simulink model "comparing_modell_MSfartoy"  (R2017b)
settings: Solver=ode45  StartTime=tstart  StopTime=tstop  RelTol=1e-3  EnableMultiTasking=on
values from neighbouring files (symbols this model uses):
  c = 0    [analyse_dynamics_v3.m]    (also in run_task_1_8.m = 1; system_identification.m = pid_matrix(i,:))
  den = data_matrix(i,2)    [system_identification.m]
  e_u_limit = 0.7    [parameters_speed_controller.m]    (also in run_task_1_8.m; system_identification.m = 100000)
  Ki_u = 0.08    [parameters_speed_controller.m]    (also in run_task_1_8.m; system_identification.m = c(4)*Ki_u_gain_list(i))
  Ki_u_est = c(4)*0.7    [system_identification.m]
  Kp_u = 80    [parameters_speed_controller.m]    (also in run_task_1_8.m; system_identification.m)
  Kp_u_est = c(2)    [system_identification.m]
  nc_gain = nc_gain_list(i)    [system_identification.m]
  num = data_matrix(i,3:4)    [system_identification.m]
  p0 = zeros(2,1)    [analyse_dynamics_v3.m]    (also in run_task_1_8.m; system_identification.m)
  psi0 = 0    [analyse_dynamics_v3.m]    (also in run_task_1_8.m; system_identification.m)
  psi_d = 0*deg2rad    (= 0)    [run_task_1_8.m]
  r0 = 0    [analyse_dynamics_v3.m]    (also in run_task_1_8.m; system_identification.m)
  r_d = 0*deg2rad    (= 0)    [run_task_1_8.m]
  tsamp = 100    [analyse_dynamics_v3.m]    (also in run_task_1_8.m = 10; system_identification.m)
  tstep = 500    [run_task_1_8.m]    (also in system_identification.m = 0)
  ustep0 = 4    [run_task_1_8.m]    (also in system_identification.m = v0(1))
  ustepend = 7    [run_task_1_8.m]    (also in system_identification.m)
  v0 = [6.63 0]'    [analyse_dynamics_v3.m]    (also in run_task_1_8.m = [4 0]'; system_identification.m = [4 0]')
  wn_u = wn_u_list(i)    [system_identification.m]
  zeta_u = 1    [parameters_speed_controller.m]    (also in system_identification.m = zeta_u_list(i))
undefined symbols (not defined in the file or in its folder): Kd_psi, Ki_psi, Ki_r, Kp_psi, Kp_r, msfartoystyring
settings Model: ExtModeAutoUpdateStatusClock=off  Creator=christh  LastModifiedBy=EllaLovise
settings DataIOCC: LimitDataPoints=on  SaveFormat=Array  SignalLoggingSaveFormat=ModelDataLogs
settings OptimizationCC: ExpressionDepthLimit=2147483647  InitFltsAndDblsToZero=on  LifeSpan=inf
settings DebuggingCC: UnderspecifiedInitializationDetection=Classic  MergeDetectMultiDrivingBlocksExec=none  SolverPrmCheckMsg=warning  FcnCallInpInsideContextMsg=warning  StateNameClashWarn=warning  SFUnexpectedBacktrackingDiag=warning  SFNoUnconditionalDefaultTransitionDiag=warning  SFExecutionAtInitializationDiag=none
settings HardwareCC: ProdBitPerPointer=32  ProdBitPerSizeT=32  ProdBitPerPtrDiffT=32  ProdLargestAtomicFloat=None  ProdIntDivRoundTo=Undefined  ProdEndianess=Unspecified  ProdWordSize=32  ProdHWDeviceType=32-bit Generic
settings ModelReferenceCC: PropagateSignalLabelsOutOfModel=off
settings CodeAppCC: StateflowObjectComments=on
settings GRTTargetCC: TargetLangStandard=C89/C90 (ANSI)  GeneratePreprocessorConditionals=Disable all  CombineOutputUpdateFcns=off  GRTInterface=on
settings ConfigComp: CovMetricSettings=dw  CovHtmlReporting=on  CovSaveCumulativeToWorkspaceVar=on  CovSaveSingleToWorkspaceVar=on  CovExternalEMLEnable=off

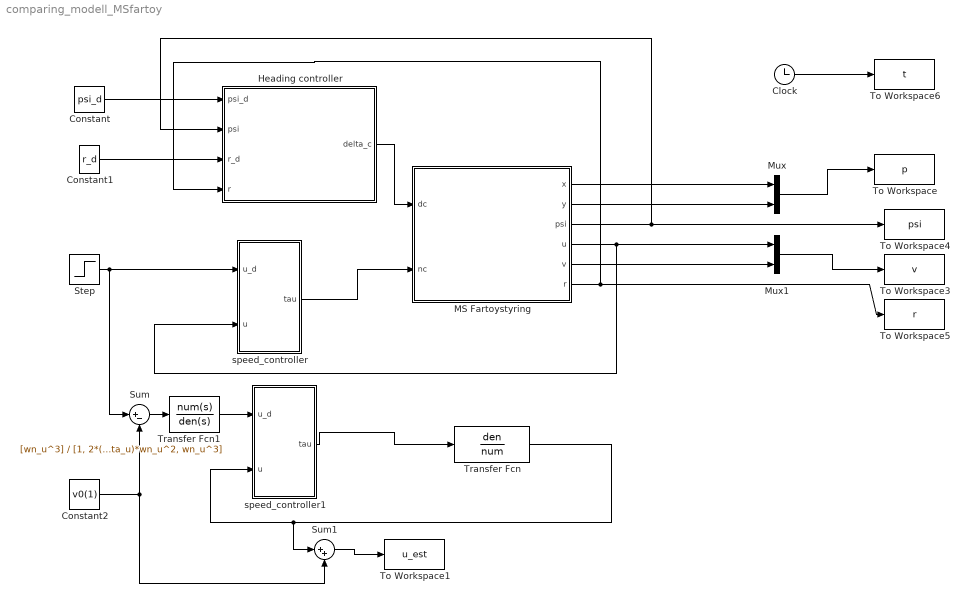
== system comparing_modell_MSfartoy ==
  Clock : Clock
  Constant : Constant  Value=psi_d
  Constant1 : Constant  Value=r_d
  Constant2 : Constant  Value=v0(1)
  Heading controller : Subsystem
  MS Fartoystyring : Subsystem  mask(MS Fartoystyring for Assignment 3 G&C){x0=p0(1), y0=p0(2), u0=v0(1), v0=v0(2), psi0=psi0, r0=r0, c=c}
      mask prompts: x0 "x(t0) (m)"; y0 "y(t0) (m)"; u0 "u(t0) (m/s)"; v0 "v(t0) (m/s)"; psi0 "psi(t0) (rad)"; r0 "r(t0) (rad/s)"; c "current (0 or 1)"
      mask help:
      | Block corresponding to Figure 1 in the assignment text. Gives the response of the ship.
      |
      | The design speed of MS Fartoystyring is u=8.23 m/s.
      |
      | Input:
      | dc: commanded rudder (rad), dmax=25*pi/180
      | nc: commanded shaft speed (rad/s), nmax=85*2*pi/60
      |
      | Output:
      | x: north pos (m)
      | y: east pos (m)
      | u: surge (m/s)
      | v: sway (m/s)
      | psi: heading (rad)
      | r: yaw (rad/s)
      mask Help: Comments, bugs and help requests can be directed to the TA. Email on course website.
  Mux : Mux  Inputs=2
  Mux1 : Mux  Inputs=2
  Step : Step  Time=tstep  Before=ustep0  After=ustepend  SampleTime=0
  Sum : Sum  Inputs=|+-
  Sum1 : Sum  Inputs=|++
  To Workspace : ToWorkspace  VariableName=p  SampleTime=tsamp
  To Workspace1 : ToWorkspace  VariableName=u_est  SampleTime=tsamp
  To Workspace3 : ToWorkspace  VariableName=v  SampleTime=tsamp
  To Workspace4 : ToWorkspace  VariableName=psi  SampleTime=tsamp
  To Workspace5 : ToWorkspace  VariableName=r  SampleTime=tsamp
  To Workspace6 : ToWorkspace  VariableName=t  SampleTime=tsamp
  Transfer Fcn : TransferFcn  Numerator=den  Denominator=num
  Transfer Fcn1 : TransferFcn  Numerator=[wn_u^3]  Denominator=[1, 2*(1+zeta_u)*wn_u , 2*(1+zeta_u)*wn_u^2, wn_u^3]
  speed_controller : Subsystem
  speed_controller1 : Subsystem
  wires:
  Clock/1 -> To Workspace6/1
  MS Fartoystyring/1(x) -> Mux/1
  MS Fartoystyring/2(y) -> Mux/2
  MS Fartoystyring/4(u) -> speed_controller/2(u), Mux1/1
  MS Fartoystyring/5(v) -> Mux1/2
  Mux/1 -> To Workspace/1
  Mux1/1 -> To Workspace3/1
  Constant1/1 -> Heading controller/3(r_d)
  MS Fartoystyring/6(r) -> Heading controller/4(r), To Workspace5/1
  MS Fartoystyring/3(psi) -> Heading controller/2(psi), To Workspace4/1
  Constant/1 -> Heading controller/1("psi_d ")
  Heading controller/1(delta_c) -> MS Fartoystyring/1(dc)
  Step/1 -> Sum/1, speed_controller/1(u_d)
  speed_controller/1(tau) -> MS Fartoystyring/2(nc)
  speed_controller1/1(tau) -> Transfer Fcn/1
  Transfer Fcn/1 -> Sum1/1, speed_controller1/2(u)
  Constant2/1 -> Sum/2, Sum1/2
  Sum1/1 -> To Workspace1/1
  Transfer Fcn1/1 -> speed_controller1/1(u_d)
  Sum/1 -> Transfer Fcn1/1

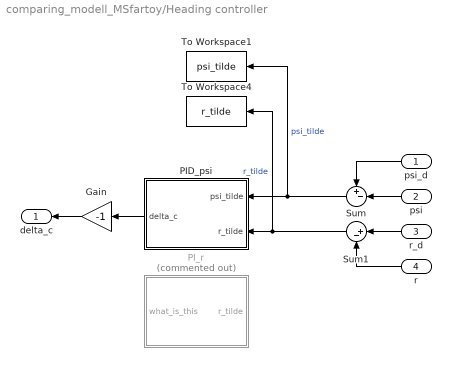
== system comparing_modell_MSfartoy/Heading controller ==
  "psi_d " : Inport
  psi : Inport  Port=2
  r_d : Inport  Port=3
  r : Inport  Port=4
  Gain : Gain  Gain=-1
  PID_psi : Subsystem
  PI_r : Subsystem  Commented=on
  Sum : Sum  Inputs=+-|
  Sum1 : Sum  Inputs=|+-
  To Workspace1 : ToWorkspace  VariableName=psi_tilde  SampleTime=tsamp
  To Workspace4 : ToWorkspace  VariableName=r_tilde  SampleTime=tsamp
  delta_c : Outport
  wires:
  psi/1 -> Sum/2
  "psi_d "/1 -> Sum/1
  Sum1/1 -> To Workspace4/1, PID_psi/2(r_tilde)  "r_tilde"
  r_d/1 -> Sum1/1
  Sum/1 -> To Workspace1/1, PID_psi/1(psi_tilde)  "psi_tilde"
  r/1 -> Sum1/2
  Gain/1 -> delta_c/1
  PID_psi/1(delta_c) -> Gain/1

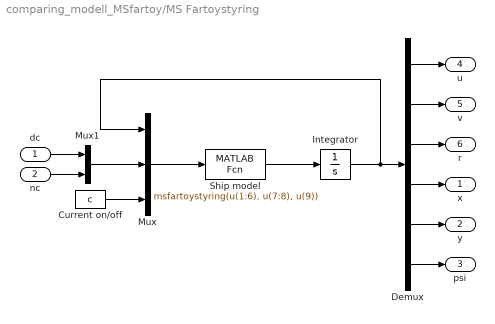
== system comparing_modell_MSfartoy/MS Fartoystyring ==
  dc : Inport
  nc : Inport  Port=2
  Current on/off : Constant  Value=c
  Demux : Demux  Outputs=6
  Integrator : Integrator  InitialCondition=[u0 v0 r0 x0 y0 psi0]'
  Mux : Mux  Inputs=3
  Mux1 : Mux  Inputs=2
  Ship model : MATLABFcn  MATLABFcn=msfartoystyring(u(1:6), u(7:8), u(9))  OutputDimensions=6
  x : Outport
  y : Outport  Port=2
  psi : Outport  Port=3
  u : Outport  Port=4
  v : Outport  Port=5
  r : Outport  Port=6
  wires:
  Integrator/1 -> Mux/1, Demux/1
  Mux1/1 -> Mux/2
  dc/1 -> Mux1/1
  nc/1 -> Mux1/2
  Demux/1 -> u/1
  Demux/2 -> v/1
  Demux/3 -> r/1
  Demux/4 -> x/1
  Demux/5 -> y/1
  Demux/6 -> psi/1
  Current on/off/1 -> Mux/3
  Ship model/1 -> Integrator/1
  Mux/1 -> Ship model/1

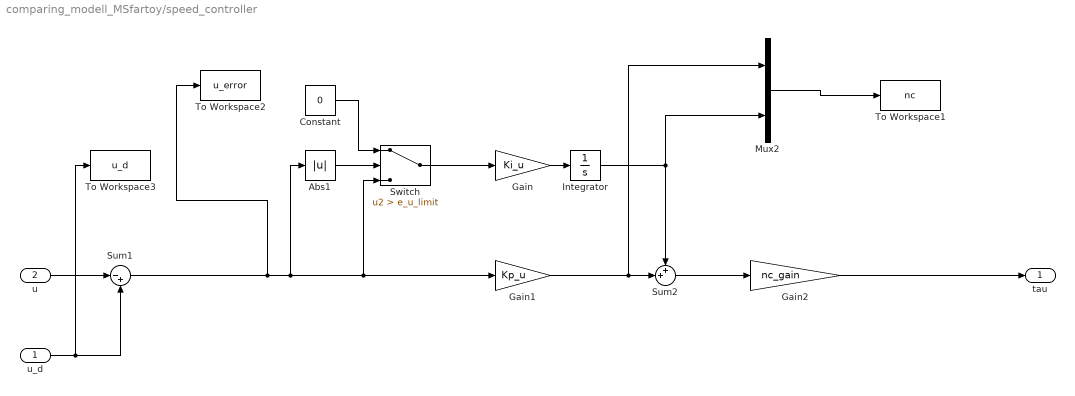
== system comparing_modell_MSfartoy/speed_controller ==
  u_d : Inport
  u : Inport  Port=2
  Abs1 : Abs
  Constant : Constant  Value=0
  Gain : Gain  Gain=Ki_u
  Gain1 : Gain  Gain=Kp_u
  Gain2 : Gain  Gain=nc_gain
  Integrator : Integrator
  Mux2 : Mux  Inputs=2
  Sum1 : Sum  Inputs=|-+
  Sum2 : Sum  Inputs=++|
  Switch : Switch  Criteria=u2 > Threshold  Threshold=e_u_limit
  To Workspace1 : ToWorkspace  VariableName=nc  SampleTime=tsamp
  To Workspace2 : ToWorkspace  VariableName=u_error  SaveFormat=Structure With Time  SampleTime=tsamp
  To Workspace3 : ToWorkspace  VariableName=u_d  SaveFormat=Structure With Time  SampleTime=tsamp
  tau : Outport
  wires:
  Gain/1 -> Integrator/1
  Mux2/1 -> To Workspace1/1
  Abs1/1 -> Switch/2
  Constant/1 -> Switch/1
  Switch/1 -> Gain/1
  Gain1/1 -> Mux2/1, Sum2/2
  Integrator/1 -> Mux2/2, Sum2/1
  u/1 -> Sum1/1
  u_d/1 -> To Workspace3/1, Sum1/2
  Sum2/1 -> Gain2/1
  Sum1/1 -> To Workspace2/1, Switch/3, Gain1/1, Abs1/1
  Gain2/1 -> tau/1

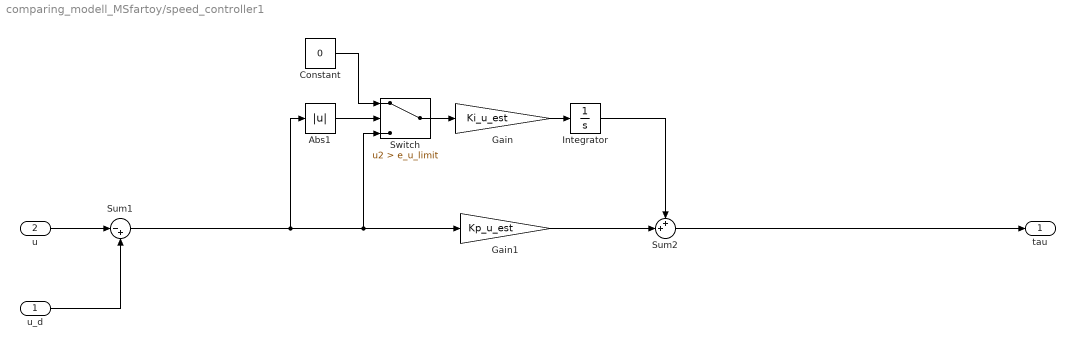
== system comparing_modell_MSfartoy/speed_controller1 ==
  u_d : Inport
  u : Inport  Port=2
  Abs1 : Abs
  Constant : Constant  Value=0
  Gain : Gain  Gain=Ki_u_est
  Gain1 : Gain  Gain=Kp_u_est
  Integrator : Integrator
  Sum1 : Sum  Inputs=|-+
  Sum2 : Sum  Inputs=++|
  Switch : Switch  Criteria=u2 > Threshold  Threshold=e_u_limit
  tau : Outport
  wires:
  Gain/1 -> Integrator/1
  Abs1/1 -> Switch/2
  Constant/1 -> Switch/1
  Switch/1 -> Gain/1
  Gain1/1 -> Sum2/2
  Integrator/1 -> Sum2/1
  u/1 -> Sum1/1
  u_d/1 -> Sum1/2
  Sum1/1 -> Switch/3, Gain1/1, Abs1/1
  Sum2/1 -> tau/1

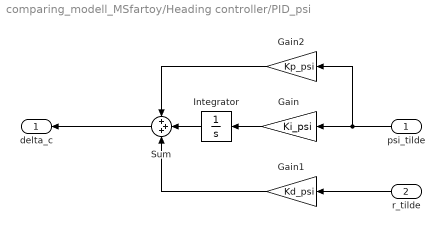
== system comparing_modell_MSfartoy/Heading controller/PID_psi ==
  psi_tilde : Inport
  r_tilde : Inport  Port=2
  Gain : Gain  Gain=Ki_psi
  Gain1 : Gain  Gain=Kd_psi
  Gain2 : Gain  Gain=Kp_psi
  Integrator : Integrator
  Sum : Sum  Inputs=+++
  delta_c : Outport
  wires:
  Gain2/1 -> Sum/1
  r_tilde/1 -> Gain1/1
  Gain1/1 -> Sum/3
  psi_tilde/1 -> Gain2/1, Gain/1
  Sum/1 -> delta_c/1
  Gain/1 -> Integrator/1
  Integrator/1 -> Sum/2

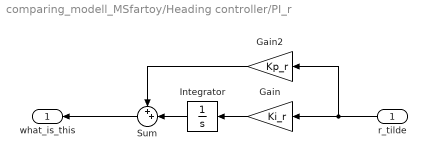
== system comparing_modell_MSfartoy/Heading controller/PI_r ==
  r_tilde : Inport
  Gain : Gain  Gain=Ki_r
  Gain2 : Gain  Gain=Kp_r
  Integrator : Integrator
  Sum : Sum  Inputs=++|
  what_is_this : Outport
  wires:
  Gain2/1 -> Sum/1
  r_tilde/1 -> Gain2/1, Gain/1
  Sum/1 -> what_is_this/1
  Gain/1 -> Integrator/1
  Integrator/1 -> Sum/2
